simulink model "GEN__S1_2"  (R2024a)
settings: Solver=VariableStepAuto  StartTime=0.0  StopTime=10.0  RelTol=1e-3
settings Model: Creator=edub  LastModifiedBy=edub

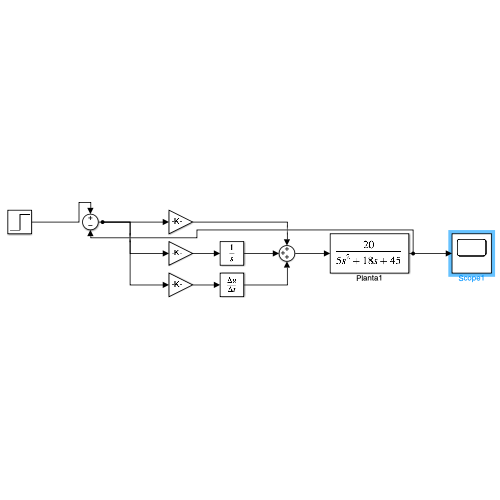
[thumbnail: Simulink's stored preview of the top-level diagram]
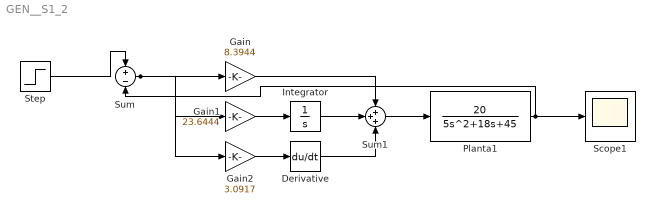
== system GEN__S1_2 ==
  Derivative : Derivative
  Gain : Gain  Gain=8.3944
  Gain1 : Gain  Gain=23.6444
  Gain2 : Gain  Gain=3.0917
  Integrator : Integrator
  Planta1 : TransferFcn  Numerator=[0 0 20]  Denominator=[5 18 45]
  Scope1 : Scope
  Step : Step  Time=0  SampleTime=0
  Sum : Sum  Inputs=+-
  Sum1 : Sum  Inputs=+++
  wires:
  Step/1 -> Sum/1
  Sum/1 -> Gain/1, Gain1/1, Gain2/1
  Gain/1 -> Sum1/1
  Gain1/1 -> Integrator/1
  Integrator/1 -> Sum1/2
  Gain2/1 -> Derivative/1
  Derivative/1 -> Sum1/3
  Sum1/1 -> Planta1/1
  Planta1/1 -> Scope1/1, Sum/2
